simulink model "Incremental_MPPT"  (R2023a)
settings: Solver=VariableStepAuto  StartTime=0.0  StopTime=2  RelTol=1e-3
undefined symbols (not defined in the file): Acid, Lead
libraries: spsSeriesRLCBranchLib x3, spsBatteryLib x1, spsDiodeLib x1, spsIGBTDiodeLib x1, spsPVArrayLib x1, simulink x1, sps_lib x1
settings Model: Creator=rahul  LastModifiedBy=SEIL

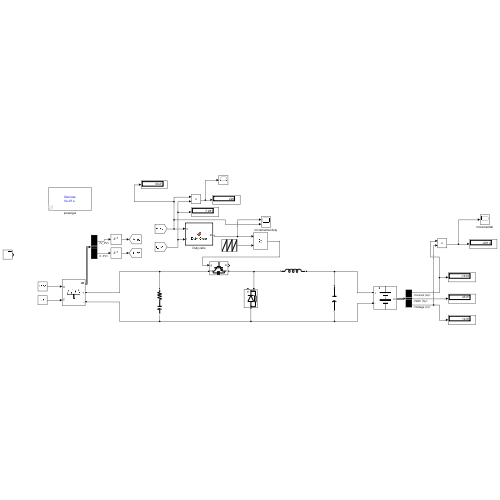
[thumbnail: Simulink's stored preview of the top-level diagram]
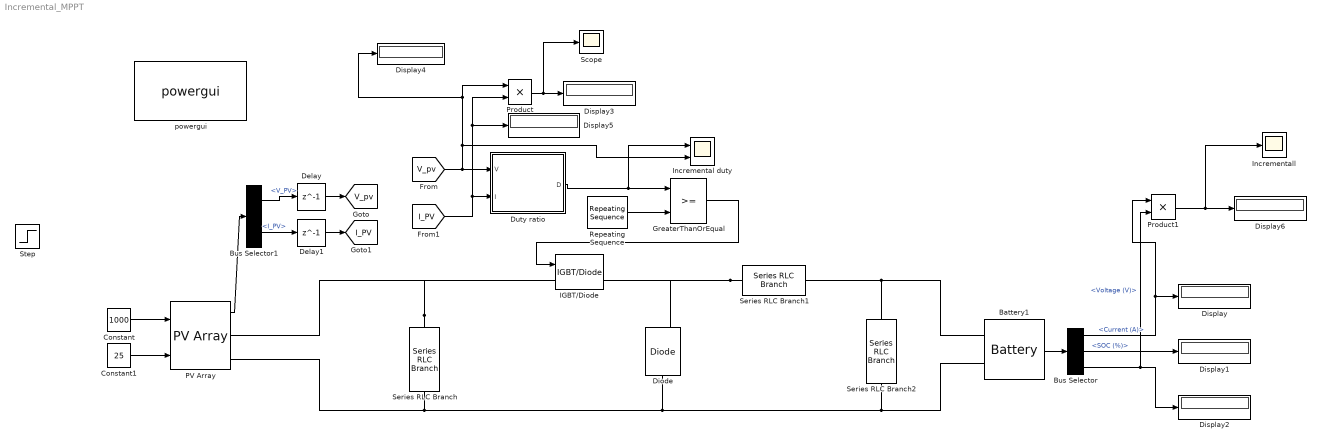
== system Incremental_MPPT ==
  Battery1 : spsBatteryLib/Battery  BatType=Lead-Acid  ShowTempParam=off  ThermalPreset=no  ShowAgeParam=off  NomV=12  NomQ=100  SOC=45  Batt_Tr=1  PresetModel=on  MaxQ=104.1667  MinV=9  FullV=13.0658  Dis_rate=20  R=0.0012  Normal_OP=31.0278  expZone="[12.2171     0.333333]"  current=[6.5 13 32.5]  Units=Time  Tci=20  NomT=20  T2=-30  MaxQ2=4.8  FullV2=7.1  Normal_OP2=5.655  expZone2="[6.58           1]"  Rca=0.6  ti=2000  Dp=0  Neq0=0  Tsim=1e6  Ta1=25  Qeol=5.4*0.9  Reol=0.013333*1.2  Char_age=[2.3478, 3]  Dis_age=[2.3478, 10]  N1=1500  N2=10500  N3=1000  N4=1400  Ta2=45  N5=950
  Bus Selector : BusSelector  OutputSignals=Current (A),SOC (%),Voltage (V)
  Bus Selector1 : BusSelector  OutputSignals=V_PV,I_PV
  Constant : Constant  Value=1000
  Constant1 : Constant  Value=25
  Delay : Delay  DelayLength=1  InitialCondition=0  SampleTime=1e-5
  Delay1 : Delay  DelayLength=1  InitialCondition=0  SampleTime=1e-5
  Diode : spsDiodeLib/Diode  Ron=0.001  Lon=0  Vf=0.8  IC=0  UseSnubber=0  Rs=500  Cs=250e-9  Measurements=on
  Display{,1..6} (7 alike) : Display
  Duty ratio : MATLAB Function  TreatAsAtomicUnit=on
  GreaterThanOrEqual : RelationalOperator  OutDataTypeStr=boolean  RndMeth=Simplest  InputSameDT=off
  IGBT/Diode : spsIGBTDiodeLib/IGBT//Diode  Ron=1e-3  Rs=1e5  Cs=inf  Measurements=on
  Incremental duty : Scope  NumInputPorts=2
  Incrementall : Scope
  PV Array : spsPVArrayLib/PV Array  Npar=1  Nser=1  PlotType=one module @ 25 deg.C & specified irradiances  S_vec="[ 1000  500  100 ]"  Temp_C_vec="[ 45 25  ]"  ModuleName=A2Peak Power POWER ON P220-6x10  PlotWhenSelected=off  Pm=219.978  Ncell=60  Voc=36.72  Isc=7.98  Vm=30.3  Im=7.26  beta_Voc_pc=-0.35  alpha_Isc_pc=0.05  beta_Voc=-0.12852  alpha_Isc=0.00399  IL=8.0041  I0=1.8441e-10  nI=0.97472  Rsh=85.0716  Rs=0.25728  RobustModel=off  RobustCellTemperature=313.3991  BAL=on  Tc=1e-6  Tfilter=5e-5
  Product : Product
  Product1 : Product
  Repeating Sequence : simulink/Sources/Repeating Sequence  rep_seq_t=[0 0.0001]  rep_seq_y=[0 1]
  Scope : Scope
  Series RLC Branch : spsSeriesRLCBranchLib/Series RLC Branch  LConnTagsString=__new0  RConnTagsString=__new0  BranchType=RC  Resistance=0.001  Inductance=0  SetiL0=off  InitialCurrent=0  Capacitance=1000e-6  Setx0=off  InitialVoltage=0  Measurements=None
  Series RLC Branch1 : spsSeriesRLCBranchLib/Series RLC Branch  LConnTagsString=__new0  RConnTagsString=__new0  BranchType=L  Resistance=1  Inductance=0.587e-3  SetiL0=off  InitialCurrent=0  Capacitance=1e-6  Setx0=off  InitialVoltage=0  Measurements=None
  Series RLC Branch2 : spsSeriesRLCBranchLib/Series RLC Branch  LConnTagsString=__new0  RConnTagsString=__new0  BranchType=C  Resistance=1  Inductance=1e-3  SetiL0=off  InitialCurrent=0  Capacitance=369.79e-6  Setx0=off  InitialVoltage=0  Measurements=None
  Step : Step  Before=100  After=1000  SampleTime=0.005
  powergui : sps_lib/powergui  Priority=1  SimulationMode=Discrete  SampleTime=50e-8  frequency=60  Iterations=50  frequencyindice=0  Pbase=100e6  ErrMax=1e-4  UnitsV=kV  UnitsW=MW  buscounter=0  FunctionMessages=off  echomessages=off  EnableUseOfTLC=off  CurrentSourceSwitches=off  DisableSnubberDevices=off  DisableRonSwitches=off  DisableVfSwitches=off  DisplayEquations=off  AutomaticDiscreteSolvers=off  SolverType=Tustin/Backward Euler (TBE)  Interpol=off  ExternalGateDelay=off  methode=off  Ts=100  x0status=blocks  SPID=on  SwTol=0  HookPort=off  NonlinearTolerance=1e-4  nMaxIteration=100  ContinueOnMaxIteration=off  RestoreLinks=warning  ResistiveCurrentMeasurement=off  Frange=[0:2:500]  Ylog=off  Xlog=on  ShowGrid=off  save=off  variable=ZData  structure=0  ZoomFFT=off  StartTime=0.0  cycles=1  DisplayStyle=1  fundamental=60  FreqAxis=off  MaxFrequency=1000  frequencyindicesteady=1  RmsSteady=1  display=off
  tag scope: I_PV=global, V_pv=global
  wires:
  [I_PV] -> Product/2, Display5/1, Duty ratio/2(I)
  Bus Selector/2 -> Display1/1  "<SOC (%)>"
  Duty ratio/1(D) -> Incremental duty/1, GreaterThanOrEqual/1
  Repeating Sequence/1 -> GreaterThanOrEqual/2
  Product/1 -> Scope/1, Display3/1
  Bus Selector/3 -> Product1/2, Display2/1  "<Voltage (V)>"
  Bus Selector1/1 -> Delay/1  "<V_PV>"
  Delay/1 -> [V_pv]
  Bus Selector/1 -> Product1/1, Display/1  "<Current (A)>"
  [V_pv] -> Display4/1, Product/1, Incremental duty/2, Duty ratio/1(V)
  GreaterThanOrEqual/1 -> IGBT/Diode/1
  Bus Selector1/2 -> Delay1/1  "<I_PV>"
  Product1/1 -> Incrementall/1, Display6/1
  PV Array/1 -> Bus Selector1/1
  Battery1/1 -> Bus Selector/1
  Delay1/1 -> [I_PV]
  Constant1/1 -> PV Array/2
  Constant/1 -> PV Array/1
  connections:
  Battery1/LConn1 -- Series RLC Branch1/RConn1 -- Series RLC Branch2/LConn1
  Battery1/LConn2 -- PV Array/RConn2 -- Series RLC Branch/RConn1 -- Diode/LConn1 -- Series RLC Branch2/RConn1
  Series RLC Branch/LConn1 -- PV Array/RConn1 -- IGBT/Diode/LConn1
  Series RLC Branch1/LConn1 -- IGBT/Diode/RConn1 -- Diode/RConn1

== matlab function Incremental_MPPT/Duty ratio ==
  data: V input; D output; I input
function D = Duty_Cycle(V,I)
Dmax = 0.95;
Dmin = 0.1;
Dinit = 0.2;
DelD = 0.00001;

persistent Vold Pold Dold Iold;

datatype = 'double';

if isempty(Vold)
	Vold = 0;
	Pold = 0;
	Iold=0;
	Dold = Dinit;
end
P = V*I;
dV = V-Vold;
dP = P-Pold;
dI = I-Iold;

if dV==0
	if dI==0
		D=Dold;
	elseif dI>0
		D=Dold-DelD;
    else 
		D=Dold+DelD;
	end
else
	if dI/dV == -I/V
		D=Dold;
	elseif dI/dV>-I/V
		D=Dold-DelD;
    else 
		D=Dold+DelD;
	end
end

if D>=Dmax || D<=Dmin
	D=Dold;
end

Dold = D;
Vold = V;
Pold = P;
Iold=I;
